simulink model "Simulation"  (R2020b)
settings: Solver=VariableStepAuto  StartTime=0.0  StopTime=36000  FixedStep=5  RelTol=1e-3
settings Model: SimulationMode=accelerator  Creator=alain  LastModifiedBy=alain

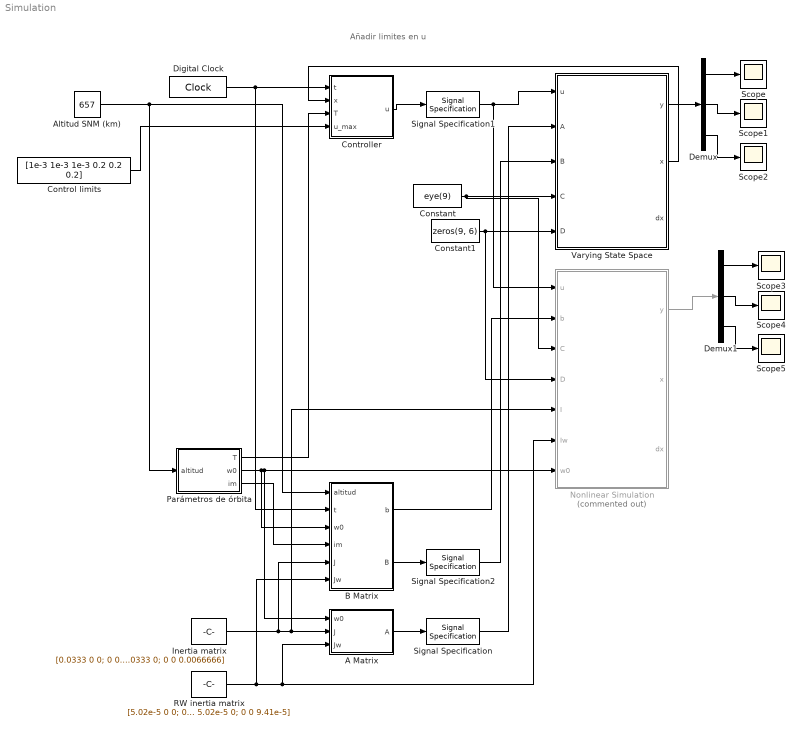
== system Simulation ==
  note: Añadir limites en u
  A Matrix : MATLAB Function  TreatAsAtomicUnit=on
  Altitud SNM (km) : Constant  Value=657
  B Matrix : MATLAB Function  TreatAsAtomicUnit=on
  Constant : Constant  Value=eye(9)
  Constant1 : Constant  Value=zeros(9, 6)
  Control limits : Constant  Value=[1e-3 1e-3 1e-3 0.2 0.2 0.2]
  Controller : MATLAB Function  TreatAsAtomicUnit=on
  Demux : Demux  Outputs=[3 3 3]
  Demux1 : Demux  Outputs=[3 3 3]
  Digital Clock : DigitalClock
  Inertia matrix : Constant  Value=[0.0333 0 0; 0 0.0333 0; 0 0 0.0066666]
  Nonlinear Simulation : Subsystem  Commented=on  AncestorBlock=cstblocks/Linear Parameter Varying/Varying State Space  mask(Varying State Space){x0=[0.4; 0.4; 0.4; 1; 1; 1; 0; 0; 0], xNames='', OutputX=on, OutputDX=on}
      mask prompts: x0 "Control:simulink:VaryingSSLabel1"; xNames "Control:simulink:VaryingSSLabel2"; OutputX "Control:simulink:VaryingSSLabel3"; OutputDX "Control:simulink:VaryingSSLabel4"
      mask help: Control:simulink:VaryingSS1
      mask init:
      | % Use exact linearization of product block
      | % pblks = find_system(gcb,'FollowLinks','on',...
      | %    'LookUnderMasks','all','SearchDepth',1,'BlockType','Product');
      | % rep = struct(...
      | %    'Specification','controllib.internal.blocks.matrixProductJacobian',...
      | %    'Type','Function',...
      | %    'ParameterNames','',...
      | %    'ParameterValues','');
      | % for i=1:numel(pblks)
      | %    set_param(pblks{i},...
      | %       'SCDEnableBlockLinearizationSpecification','on',...
      | %       'SCDBlockLinearizationSpecification',rep)
      | % end
      | SimStatus = get_param(bdroot,'SimulationStatus');
      | if any(strcmp(SimStatus,{'initializing','updating','stopped'}))
      |    varyingBlockMask('ss',gcb,OutputX,OutputDX)
      | end
      mask Help: eval('ctrlguihelp(''VaryingSSCT'');')
      mask DialogControl x0 Prompt: Initial conditions:
      mask DialogControl xNames Prompt: State names (e.g., 'position'):
      mask DialogControl OutputX Prompt: Output states
      mask DialogControl OutputDX Prompt: Output state derivatives
      mask Display:
      | port_label('input', 1, 'u')
      | port_label('input', 2, 'b')
      | port_label('input', 3, 'C')
      | port_label('input', 4, 'D')
      | port_label('input', 5, 'I')
      | port_label('input', 6, 'Iw')
      | port_label('input', 7, 'w0')
      | port_label('output', 1, 'y')
      | next_ = 2;
      | if OutputX
      |    port_label('output', next_, 'x')
      |    next_ = next_+1;
      | end
      | if OutputDX
      |    port_label('output', next_, 'dx')
      |    next_ = next_+1;
      | end
      | text(0.5,0.65,'dx = f(x)',...
      |    'horizontalAlignment', 'center','texmode','on')
      | text(0.5,0.35,'y = C x + D u',...
      |    'horizontalAlignment', 'center','texmode','on')
  Parámetros de órbita : MATLAB Function  TreatAsAtomicUnit=on
  RW inertia matrix : Constant  Value=[5.02e-5 0 0; 0 5.02e-5 0; 0 0 9.41e-5]
  Scope{,1..5} (6 alike) : Scope
  Signal Specification : SignalSpecification  Dimensions=[9 9]
  Signal Specification1 : SignalSpecification  Dimensions=[6 1]
  Signal Specification2 : SignalSpecification  Dimensions=[9 6]
  Varying State Space : Subsystem  AncestorBlock=cstblocks/Linear Parameter Varying/Varying State Space  mask(Varying State Space){x0=[0.4; 0.4; 0.4; 1; 1; 1; 0; 0; 0], xNames='', OutputX=on, OutputDX=on}
      mask prompts: x0 "Control:simulink:VaryingSSLabel1"; xNames "Control:simulink:VaryingSSLabel2"; OutputX "Control:simulink:VaryingSSLabel3"; OutputDX "Control:simulink:VaryingSSLabel4"
      mask help: Control:simulink:VaryingSS1
      mask init: same as Simulation/Nonlinear Simulation
      mask Help: eval('ctrlguihelp(''VaryingSSCT'');')
      mask DialogControl x0 Prompt: Initial conditions:
      mask DialogControl xNames Prompt: State names (e.g., 'position'):
      mask DialogControl OutputX Prompt: Output states
      mask DialogControl OutputDX Prompt: Output state derivatives
      mask Display:
      | port_label('input', 1, 'u')
      | port_label('input', 2, 'A')
      | port_label('input', 3, 'B')
      | port_label('input', 4, 'C')
      | port_label('input', 5, 'D')
      | port_label('output', 1, 'y')
      | next_ = 2;
      | if OutputX
      |    port_label('output', next_, 'x')
      |    next_ = next_+1;
      | end
      | if OutputDX
      |    port_label('output', next_, 'dx')
      |    next_ = next_+1;
      | end
      | text(0.5,0.65,'dx = A x + B u',...
      |    'horizontalAlignment', 'center','texmode','on')
      | text(0.5,0.35,'y = C x + D u',...
      |    'horizontalAlignment', 'center','texmode','on')
  wires:
  B Matrix/1(b) -> Nonlinear Simulation/2(b)
  Controller/1(u) -> Signal Specification1/1
  Signal Specification1/1 -> Varying State Space/1(u), Nonlinear Simulation/1(u)
  Varying State Space/1(y) -> Demux/1
  A Matrix/1(A) -> Signal Specification/1
  Constant/1 -> Varying State Space/4(C), Nonlinear Simulation/3(C)
  Demux/1 -> Scope/1
  Demux/2 -> Scope1/1
  Parámetros de órbita/1(T) -> Controller/3(T)
  Signal Specification2/1 -> Varying State Space/3(B)
  Demux/3 -> Scope2/1
  Signal Specification/1 -> Varying State Space/2(A)
  B Matrix/2(B) -> Signal Specification2/1
  Parámetros de órbita/3(im) -> B Matrix/4(im)
  Varying State Space/2(x) -> Controller/2(x)
  Altitud SNM (km)/1 -> B Matrix/1(altitud), Parámetros de órbita/1(altitud)
  Parámetros de órbita/2(w0) -> A Matrix/1(w0), Nonlinear Simulation/7(w0), B Matrix/3(w0)
  RW inertia matrix/1 -> A Matrix/3(Jw), Nonlinear Simulation/6(Iw), B Matrix/6(Jw)
  Digital Clock/1 -> B Matrix/2(t), Controller/1(t)
  Inertia matrix/1 -> A Matrix/2(J), Nonlinear Simulation/5(I), B Matrix/5(J)
  Constant1/1 -> Varying State Space/5(D), Nonlinear Simulation/4(D)
  Demux1/3 -> Scope5/1
  Demux1/2 -> Scope4/1
  Demux1/1 -> Scope3/1
  Nonlinear Simulation/1(y) -> Demux1/1
  Control limits/1 -> Controller/4(u_max)

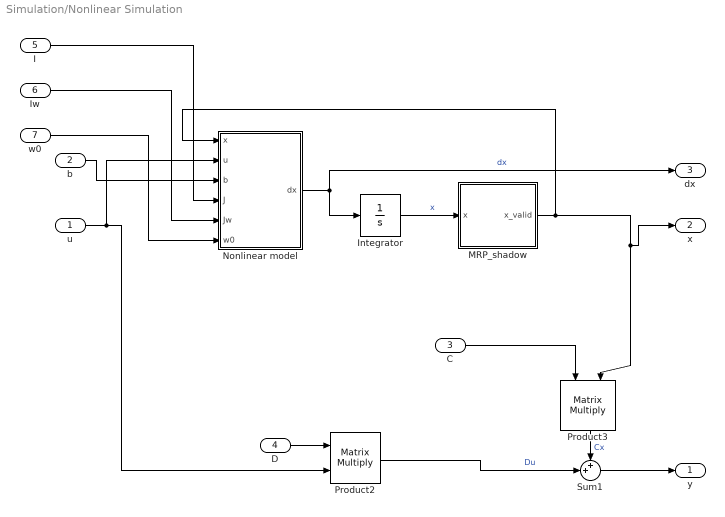
== system Simulation/Nonlinear Simulation ==
  u : Inport
  b : Inport  Port=2
  C : Inport  Port=3
  D : Inport  Port=4
  I : Inport  Port=5
  Iw : Inport  Port=6
  w0 : Inport  Port=7
  Integrator : Integrator  InitialCondition=x0  ContinuousStateAttributes=xNames
  MRP_shadow : MATLAB Function  TreatAsAtomicUnit=on
  Nonlinear model : MATLAB Function  TreatAsAtomicUnit=on
  Product2 : Product  SCDEnableBlockLinearizationSpecification=on  Multiplication=Matrix(*)
  Product3 : Product  SCDEnableBlockLinearizationSpecification=on  Multiplication=Matrix(*)
  Sum1 : Sum  Inputs=++|
  y : Outport  VectorParamsAs1DForOutWhenUnconnected=off
  x : Outport  Port=2  VectorParamsAs1DForOutWhenUnconnected=off
  dx : Outport  Port=3  VectorParamsAs1DForOutWhenUnconnected=off
  wires:
  C/1 -> Product3/1
  D/1 -> Product2/1
  u/1 -> Product2/2, Nonlinear model/2(u)
  Sum1/1 -> y/1
  Product2/1 -> Sum1/2  "Du"
  Product3/1 -> Sum1/1  "Cx"
  Nonlinear model/1(dx) -> dx/1, Integrator/1  "dx"
  Integrator/1 -> MRP_shadow/1(x)  "x"
  MRP_shadow/1(x_valid) -> Nonlinear model/1(x), Product3/2, x/1
  b/1 -> Nonlinear model/3(b)
  w0/1 -> Nonlinear model/6(w0)
  Iw/1 -> Nonlinear model/5(Jw)
  I/1 -> Nonlinear model/4(J)

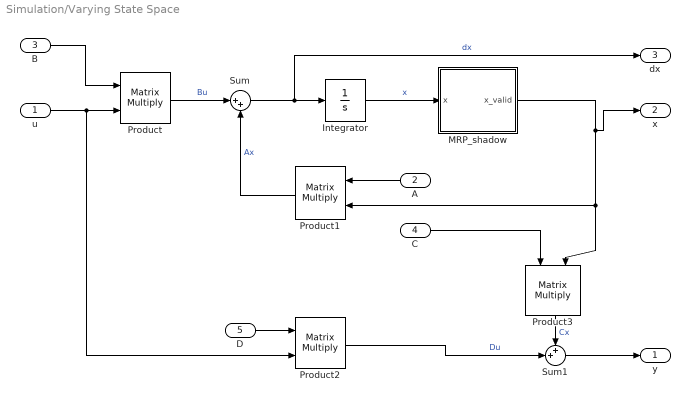
== system Simulation/Varying State Space ==
  u : Inport
  A : Inport  Port=2
  B : Inport  Port=3
  C : Inport  Port=4
  D : Inport  Port=5
  Integrator : Integrator  InitialCondition=x0  ContinuousStateAttributes=xNames
  MRP_shadow : MATLAB Function  TreatAsAtomicUnit=on
  Product{,1..3} (4 alike) : Product  SCDEnableBlockLinearizationSpecification=on  Multiplication=Matrix(*)
  Sum : Sum  Inputs=|++
  Sum1 : Sum  Inputs=++|
  y : Outport  VectorParamsAs1DForOutWhenUnconnected=off
  x : Outport  Port=2  VectorParamsAs1DForOutWhenUnconnected=off
  dx : Outport  Port=3  VectorParamsAs1DForOutWhenUnconnected=off
  wires:
  C/1 -> Product3/1
  D/1 -> Product2/1
  u/1 -> Product2/2, Product/2
  A/1 -> Product1/1
  Product1/1 -> Sum/2  "Ax"
  B/1 -> Product/1
  Sum1/1 -> y/1
  Product2/1 -> Sum1/2  "Du"
  Product3/1 -> Sum1/1  "Cx"
  Sum/1 -> Integrator/1, dx/1  "dx"
  Product/1 -> Sum/1  "Bu"
  Integrator/1 -> MRP_shadow/1(x)  "x"
  MRP_shadow/1(x_valid) -> Product1/2, Product3/2, x/1

== matlab function Simulation/Parámetros de órbita ==
  data: altitud input; T output; w0 output; im output
function [T, w0, im]= OP(altitud)

mu = 3.986005e14;

a = 6371000+altitud*1000;
T = 2 * pi * sqrt(a^3/mu);
w0 = 2 * pi / T;

im = ((altitud+2.3850e+04)/(57.3*(900-500)/(99-97.4)));

== matlab function Simulation/Controller ==
  data: t input; u output; x input; T input; u_max input
function u = Controller(t, x, T, u_max)
    data = load('Gains.mat');
    Ks = data.Ks;
    N = size(Ks);

    T_frac=T/N(3);
    t = t - floor(t/T)*T;
    n = floor(t/ T_frac)+1;

    K = Ks(:, :, n);
    u = - K * x;
    for i = 1:6
        if u(i) > u_max(i)
            u(i) = u_max(i);
        elseif u(i) < -u_max(i)
            u(i) = -u_max(i);
        end
        
    end

== matlab function Simulation/A Matrix ==
  data: w0 input; A output; J input; Jw input
function A = State(w0, J, Jw)
    W_RSW = [0, -w0, 0];
    A11 = -0.5*CrossMatrix(W_RSW)  * (4 * CrossMatrix(W_RSW) + 16 * eye(3));

    A12 = .25 * eye(3);

    A21 = [16 * w0 ^ 2 * (J(3, 3) - J(2, 2))/J(1, 1), 0, 0;
        0, 12 * w0 ^ 2 *(J(3, 3) - J(1, 1))/J(2, 2), 0;
        0, 0, 4 * w0 ^ 2 * (J(1, 1) - J(2, 2))/J(3, 3)];

    A22 = [0 0 w0 * (J(1, 1) - J(2, 2) + J(3, 3)) / J(1, 1);
        0 0 0;
        -w0 * (J(1, 1) - J(2, 2) + J(3, 3)) / J(3, 3) 0 0];

    A23 = [0 0 w0 * Jw(3, 3) /J(1, 1);
        0 0 0;
        -w0 * Jw(1, 1) / J(3, 3) 0 0];

    A = [A11 A12 zeros(3);
        A21 A22 A23;
        zeros(3) zeros(3) zeros(3)];

== matlab function Simulation/B Matrix ==
  data: b output; altitud input; B output; t input; w0 input; im input; J input; Jw input
function [b, B]= Control(altitud, t, w0, im, J, Jw)
    a = 6371000+altitud*1000;
    mf = 7.9e15;
    b = mf / a ^ 3 * [cos(w0 * t) * sin(im);
            -cos(im);
            2 * sin(w0 * t) * sin(im)];

    B = [zeros(3) zeros(3)
        inv(J), -inv(J) * CrossMatrix(b);
        -inv(Jw) zeros(3)];

== matlab function Simulation/Varying State Space/MRP_shadow ==
  data: x input; x_valid output
function x_valid = MRP_shadow(x)

s = x(1:3);
S = norm(s);

if S>=1
    s = -s/S^2;
end

x(1:3) = s;
x_valid = x;

== matlab function Simulation/Nonlinear Simulation/MRP_shadow ==
  data: x input; x_valid output
function x_valid = MRP_shadow(x)

s = x(1:3);
S = norm(s);

if S>=1
    s = -s/S^2;
end

x(1:3) = s;
x_valid = x;

== matlab function Simulation/Nonlinear Simulation/Nonlinear model ==
  data: x input; u input; dx output; b input; J input; Jw input; w0 input
function dx = model(x, u, b, J, Jw, w0)
    s = x(1:3);
    w = x(4:6);
    O = x(7:9);
    
    tw = u(1:3);
    m = u(4:6);
    
    w_RSW = [0; -w0; 0];
    
    C = eye(3) + (8 * CrossMatrix(s)*CrossMatrix(s)-4*(1-(s'*s)^2)*CrossMatrix(s))/ (1+(s'*s)^2)^2;
    w_RSW_b = C * w_RSW;
    
    tg = 3 * w0^2 * cross(C(:,3), J*C(:,3));
    Idw = cross(J*w, w_RSW_b)-cross((w+w_RSW_b), J*(w + w_RSW_b)+ Jw*O) + tw + tg - CrossMatrix(b)*m;
    
    ds = (1/4) * ((1 - s' * s)* eye(3) + 2 * CrossMatrix(s) + 2 * (s * s')) * w;
    dw = J\Idw;
    dO = -inv(Jw) * tw;
    dx = [ds; dw; dO];
